simulink model "YCbCrWorking"  (Simulink 7.7)
settings: Solver=ode45  StartTime=0.0  StopTime=10.0  RelTol=1e-3
undefined symbols (not defined in the file or in its folder): gray
libraries: vipsnks x2, vipconversions x1, dspsrcs4 x1
settings Model: Creator=katsikas  LastModifiedBy=katsikas

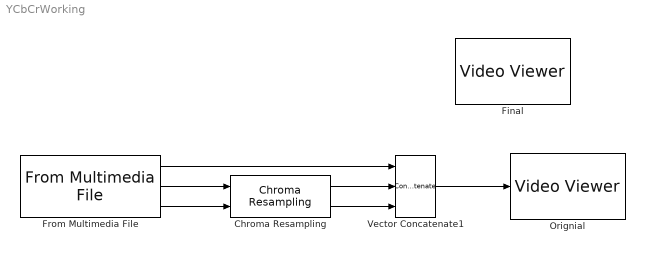
== system YCbCrWorking ==
  Chroma Resampling : vipconversions/Chroma Resampling  resampling=4:2:2 to 4:4:4  interpolation=linear  antialiasing=Default  hcoeff=[0.2 0.6 0.2]  vcoeff=[0.5 0.5]  isInputTransposed=off
  Final : vipsnks/Video Viewer  inputType=Obsolete7b  imagePorts=One multidimensional signal  useColorMap=off  colormapValue=gray(256)  specRange=off  minInputVal=0  maxInputVal=255  FigPos=[635 674 410 300]  AxisZoom=on  trueSizedOnce=on  OpenAtMdlStart=on
  From Multimedia File : dspsrcs4/From Multimedia File  inputFilename=vipmen.avi  loop=on  numPlays=inf  outputStreams=Video only  videoDataType=double  audioDataType=int16  inheritSampleTime=on  userDefinedSampleTime=1/30  noAudioOutput=off  isIntensityVideo=off  fourcc=YCbCr 4:2:2  colorVideoFormat=Separate color signals  outputEOF=off  dataOrg=Column-major  audioFrameSize=1024  computeAudioFrameSize=off
  Orignial : vipsnks/Video Viewer  inputType=Obsolete7b  imagePorts=One multidimensional signal  useColorMap=off  colormapValue=gray(256)  specRange=off  minInputVal=0  maxInputVal=255  FigPos=[634 644 410 300]  AxisZoom=on  trueSizedOnce=on  OpenAtMdlStart=on
  Vector Concatenate1 : Concatenate  NumInputs=3  Mode=Multidimensional array  ConcatenateDimension=3
  wires:
  Vector Concatenate1/1 -> Orignial/1
  Chroma Resampling/2 -> Vector Concatenate1/3
  Chroma Resampling/1 -> Vector Concatenate1/2
  From Multimedia File/1 -> Vector Concatenate1/1
  From Multimedia File/2 -> Chroma Resampling/1
  From Multimedia File/3 -> Chroma Resampling/2
